simulink model "voltera"  (R2014b)
settings: Solver=ode4  StartTime=0.0  StopTime=10.0  FixedStep=0.01  RelTol=1e-3
values from neighbouring files (symbols this model uses):
  a = double(s)    [wprowadzenie.m]    (also in wprowadzenie2.m = int16(rand*3))
  b = 20.03e-3    (= 0.02003)    [wprowadzenie.m]
  c = 1+3i    [wprowadzenie.m]
undefined symbols (not defined in the file or in its folder): d
settings Model: Creator=podstawy  LastModifiedBy=podstawy

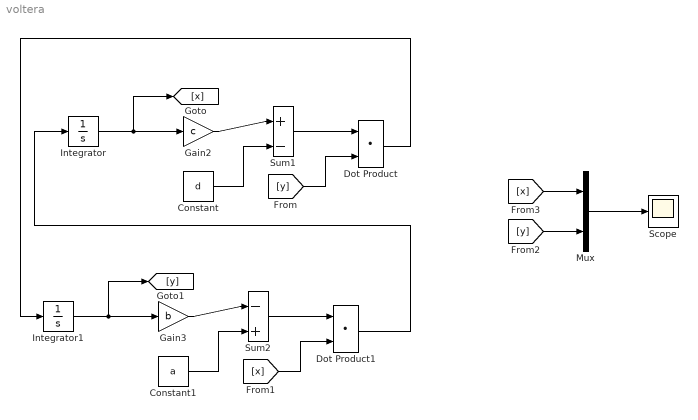
== system voltera ==
  Constant : Constant  Value=d
  Constant1 : Constant  Value=a
  Dot Product : DotProduct  InputSameDT=on  OutDataTypeStr=Inherit: Inherit via internal rule
  Dot Product1 : DotProduct  InputSameDT=on  OutDataTypeStr=Inherit: Inherit via internal rule
  Gain2 : Gain  Gain=c
  Gain3 : Gain  Gain=b
  Integrator : Integrator  InitialCondition=100
  Integrator1 : Integrator  InitialCondition=10
  Mux : Mux  Inputs=2
  Scope : Scope
  Sum1 : Sum  Inputs=|+-
  Sum2 : Sum  Inputs=|-+
  wires:
  Integrator/1 -> [x], Gain2/1
  Gain2/1 -> Sum1/1
  Constant/1 -> Sum1/2
  Sum1/1 -> Dot Product/1
  [y] -> Dot Product/2
  Integrator1/1 -> [y], Gain3/1
  Gain3/1 -> Sum2/1
  Constant1/1 -> Sum2/2
  Sum2/1 -> Dot Product1/1
  [x] -> Dot Product1/2
  Dot Product/1 -> Integrator1/1
  Dot Product1/1 -> Integrator/1
  [x] -> Mux/1
  [y] -> Mux/2
  Mux/1 -> Scope/1
